simulink model "c_lab6_sim"  (R2020b)
settings: Solver=VariableStepAuto  StartTime=0.0  StopTime=10  RelTol=1e-3
settings Model: Creator=musa oğural  LastModifiedBy=musa oğural

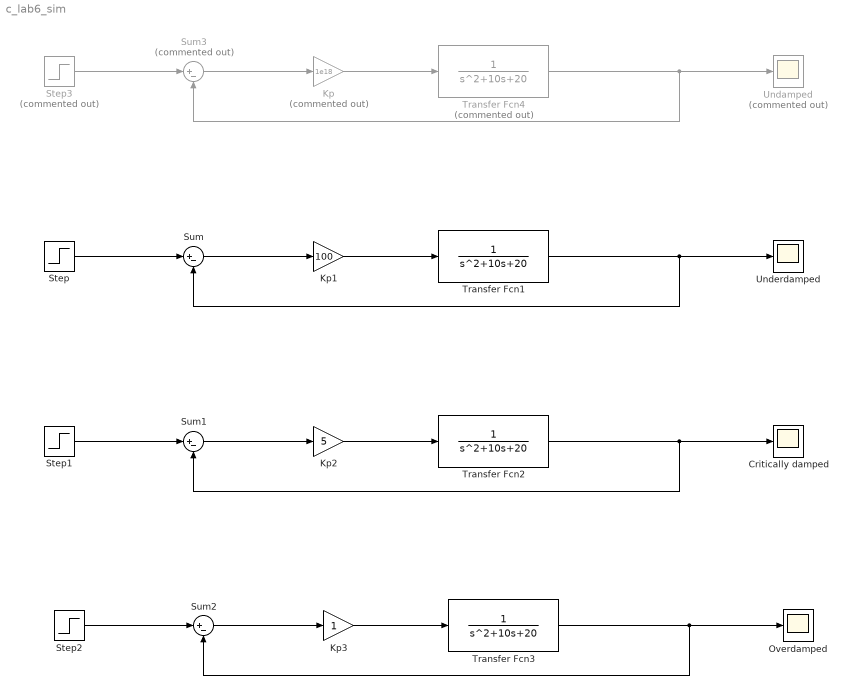
== system c_lab6_sim ==
  Critically damped : Scope
  Kp : Gain  Commented=on  Gain=1e18
  Kp1 : Gain  Gain=100
  Kp2 : Gain  Gain=5
  Kp3 : Gain
  Overdamped : Scope
  Step : Step  Time=0  SampleTime=0
  Step1 : Step  Time=0  SampleTime=0
  Step2 : Step  Time=0  SampleTime=0
  Step3 : Step  Commented=on  Time=0  SampleTime=0
  Sum : Sum  Inputs=|+-
  Sum1 : Sum  Inputs=|+-
  Sum2 : Sum  Inputs=|+-
  Sum3 : Sum  Commented=on  Inputs=|+-
  Transfer Fcn1 : TransferFcn  Denominator=[1 10 20]
  Transfer Fcn2 : TransferFcn  Denominator=[1 10 20]
  Transfer Fcn3 : TransferFcn  Denominator=[1 10 20]
  Transfer Fcn4 : TransferFcn  Commented=on  Denominator=[1 10 20]
  Undamped : Scope  Commented=on
  Underdamped : Scope
  wires:
  Kp1/1 -> Transfer Fcn1/1
  Sum/1 -> Kp1/1
  Step/1 -> Sum/1
  Transfer Fcn1/1 -> Sum/2, Underdamped/1
  Step1/1 -> Sum1/1
  Transfer Fcn2/1 -> Sum1/2, Critically damped/1
  Kp2/1 -> Transfer Fcn2/1
  Sum1/1 -> Kp2/1
  Step2/1 -> Sum2/1
  Transfer Fcn3/1 -> Sum2/2, Overdamped/1
  Kp3/1 -> Transfer Fcn3/1
  Sum2/1 -> Kp3/1
  Step3/1 -> Sum3/1
  Transfer Fcn4/1 -> Sum3/2, Undamped/1
  Kp/1 -> Transfer Fcn4/1
  Sum3/1 -> Kp/1
